simulink model "tank_based_bi_teleop_pp_kalman"  (R2020b)
settings: Solver=FixedStepAuto  StartTime=0.0  StopTime=30  FixedStep=Ts  RelTol=1e-3
values from neighbouring files (symbols this model uses):
  A = 1    [four_channel_bilateral_teleoperation_kalman_params.m]    (also in four_channel_bilateral_teleoperation_params.m; kalman_test.m = [1 Ts Ts^2/2; 0 1 Ts; 0 0 1]; recursive_estimation.m = [1 Ts Ts^2/2; 0 1 Ts; 0 0 1]; scattering_based_bi_teleop_pf_kalman_params.m)
  alpha = 0.1    [tank_based_bi_teleop_pf_kalman.m]    (also in tank_based_bi_teleop_pf_params.m; tank_based_bi_teleop_pp_kalman.m = 1; tank_based_bi_teleop_pp_params.m = 1)
  Be = 100    [four_channel_bilateral_teleoperation_architecture_params.m]    (also in four_channel_bilateral_teleoperation_kalman_params.m = 0; four_channel_bilateral_teleoperation_params.m = 0; scattering_based_bi_teleop_pf_kalman_params.m = 10; scattering_based_bi_teleop_pf_params.m = 10)
  beta = 0.01    [tank_based_bi_teleop_pf_kalman.m]    (also in tank_based_bi_teleop_pf_params.m; tank_based_bi_teleop_pp_kalman.m = 0.2; tank_based_bi_teleop_pp_params.m = 0.2)
  Bh = 70    [four_channel_bilateral_teleoperation_architecture_params.m]    (also in four_channel_bilateral_teleoperation_kalman_params.m; four_channel_bilateral_teleoperation_params.m; scattering_based_bi_teleop_pf_kalman_params.m = 1.5; scattering_based_bi_teleop_pf_params.m = 1.5)
  Bm = 1    [four_channel_bilateral_teleoperation_architecture_params.m]    (also in four_channel_bilateral_teleoperation_kalman_params.m = 0.8; four_channel_bilateral_teleoperation_params.m = 0.8; scattering_based_bi_teleop_pf_kalman_params.m = 0; scattering_based_bi_teleop_pp_kalman_params.m = 15)
  Bs = 1    [four_channel_bilateral_teleoperation_architecture_params.m]    (also in four_channel_bilateral_teleoperation_kalman_params.m = 3.2; four_channel_bilateral_teleoperation_params.m = 3.2; scattering_based_bi_teleop_pf_kalman_params.m = 40; scattering_based_bi_teleop_pf_params.m = 3)
  delay = 10    [scattering_based_bi_teleop_pf_kalman_params.m]    (also in scattering_based_bi_teleop_pf_params.m = 1; scattering_based_bi_teleop_pp_kalman_params.m = 1; scattering_based_bi_teleop_pp_params.m = 1; tank_based_bi_teleop_pf_kalman.m)
  Dm = 5    [four_channel_bilateral_teleoperation_architecture_params.m]    (also in four_channel_bilateral_teleoperation_kalman_params.m = 0; four_channel_bilateral_teleoperation_params.m = 0; scattering_based_bi_teleop_pf_kalman_params.m = 0; scattering_based_bi_teleop_pf_params.m = 0)
  Ds = 10    [four_channel_bilateral_teleoperation_architecture_params.m]    (also in four_channel_bilateral_teleoperation_kalman_params.m = 0; four_channel_bilateral_teleoperation_params.m = 0; scattering_based_bi_teleop_pf_kalman_params.m = 0; scattering_based_bi_teleop_pf_params.m = 0)
  Fc = 1    [four_channel_bilateral_teleoperation_kalman_params.m]    (also in four_channel_bilateral_teleoperation_params.m; kalman_test.m = 10; scattering_based_bi_teleop_pf_kalman_params.m = 0.1; scattering_based_bi_teleop_pf_params.m)
  Fip = 1    [four_channel_bilateral_teleoperation_kalman_params.m]    (also in four_channel_bilateral_teleoperation_params.m; scattering_based_bi_teleop_pf_kalman_params.m = 5; scattering_based_bi_teleop_pf_params.m; scattering_based_bi_teleop_pp_kalman_params.m = 5)
  h_limit = 1    [tank_based_bi_teleop_pf_kalman.m]    (also in tank_based_bi_teleop_pf_params.m = 0.5; tank_based_bi_teleop_pp_kalman.m; tank_based_bi_teleop_pp_params.m = 1.5)
  H_master_init = 1    [tank_based_bi_teleop_pf_kalman.m]    (also in tank_based_bi_teleop_pf_params.m = 0; tank_based_bi_teleop_pp_kalman.m = 5; tank_based_bi_teleop_pp_params.m = 0)
  H_slave_init = 1    [tank_based_bi_teleop_pf_kalman.m]    (also in tank_based_bi_teleop_pf_params.m = 0; tank_based_bi_teleop_pp_kalman.m = 5; tank_based_bi_teleop_pp_params.m = 0)
  Ih = 2    [scattering_based_bi_teleop_pf_kalman_params.m]    (also in scattering_based_bi_teleop_pp_kalman_params.m; tank_based_bi_teleop_pf_kalman.m; tank_based_bi_teleop_pf_params.m; tank_based_bi_teleop_pp_kalman.m)
  Je = 0    [four_channel_bilateral_teleoperation_architecture_params.m]    (also in four_channel_bilateral_teleoperation_kalman_params.m; four_channel_bilateral_teleoperation_params.m; scattering_based_bi_teleop_pf_kalman_params.m; scattering_based_bi_teleop_pf_params.m)
  Jh = 0.5    [four_channel_bilateral_teleoperation_architecture_params.m]    (also in four_channel_bilateral_teleoperation_kalman_params.m; four_channel_bilateral_teleoperation_params.m; scattering_based_bi_teleop_pf_kalman_params.m = 0; scattering_based_bi_teleop_pf_params.m = 0.05)
  Ke = 200    [four_channel_bilateral_teleoperation_architecture_params.m]    (also in four_channel_bilateral_teleoperation_kalman_params.m = 50; four_channel_bilateral_teleoperation_params.m; scattering_based_bi_teleop_pf_kalman_params.m; scattering_based_bi_teleop_pf_params.m)
  Kh = 2000    [four_channel_bilateral_teleoperation_architecture_params.m]    (also in four_channel_bilateral_teleoperation_kalman_params.m; four_channel_bilateral_teleoperation_params.m; scattering_based_bi_teleop_pf_kalman_params.m = 1; scattering_based_bi_teleop_pf_params.m = 0)
  Km = 1    [four_channel_bilateral_teleoperation_architecture_params.m]    (also in four_channel_bilateral_teleoperation_kalman_params.m; four_channel_bilateral_teleoperation_params.m; scattering_based_bi_teleop_pf_kalman_params.m = 0; scattering_based_bi_teleop_pp_kalman_params.m = 10)
  Ks = 1    [four_channel_bilateral_teleoperation_architecture_params.m]    (also in four_channel_bilateral_teleoperation_kalman_params.m = 4; four_channel_bilateral_teleoperation_params.m = 4; scattering_based_bi_teleop_pf_kalman_params.m = 50; scattering_based_bi_teleop_pf_params.m = 110)
  Mm = 0.5    [four_channel_bilateral_teleoperation_architecture_params.m]    (also in four_channel_bilateral_teleoperation_kalman_params.m; four_channel_bilateral_teleoperation_params.m; scattering_based_bi_teleop_pf_kalman_params.m; scattering_based_bi_teleop_pf_params.m)
  Ms = 2    [four_channel_bilateral_teleoperation_architecture_params.m]    (also in four_channel_bilateral_teleoperation_kalman_params.m; four_channel_bilateral_teleoperation_params.m; scattering_based_bi_teleop_pf_kalman_params.m; scattering_based_bi_teleop_pf_params.m)
  Ph = 2000    [four_channel_bilateral_teleoperation_kalman_params.m]    (also in four_channel_bilateral_teleoperation_params.m = 20100; scattering_based_bi_teleop_pf_kalman_params.m = 5; scattering_based_bi_teleop_pf_params.m = 23; scattering_based_bi_teleop_pp_kalman_params.m = 6)
  Ts = 0.001    [four_channel_bilateral_teleoperation_kalman_params.m]    (also in four_channel_bilateral_teleoperation_params.m; kalman_test.m; recursive_estimation.m; scattering_based_bi_teleop_pf_kalman_params.m)
  VarianceVelocities = 0.001    [four_channel_bilateral_teleoperation_kalman_params.m]    (also in scattering_based_bi_teleop_pf_kalman_params.m = 1e-05; scattering_based_bi_teleop_pp_kalman_params.m = 1e-05; scattering_based_bilateral_teleoperation_pp_params.m = 1e-06; tank_based_bi_teleop_pf_kalman.m = 1e-05)
settings Model: Creator=anuj  LastModifiedBy=filippo

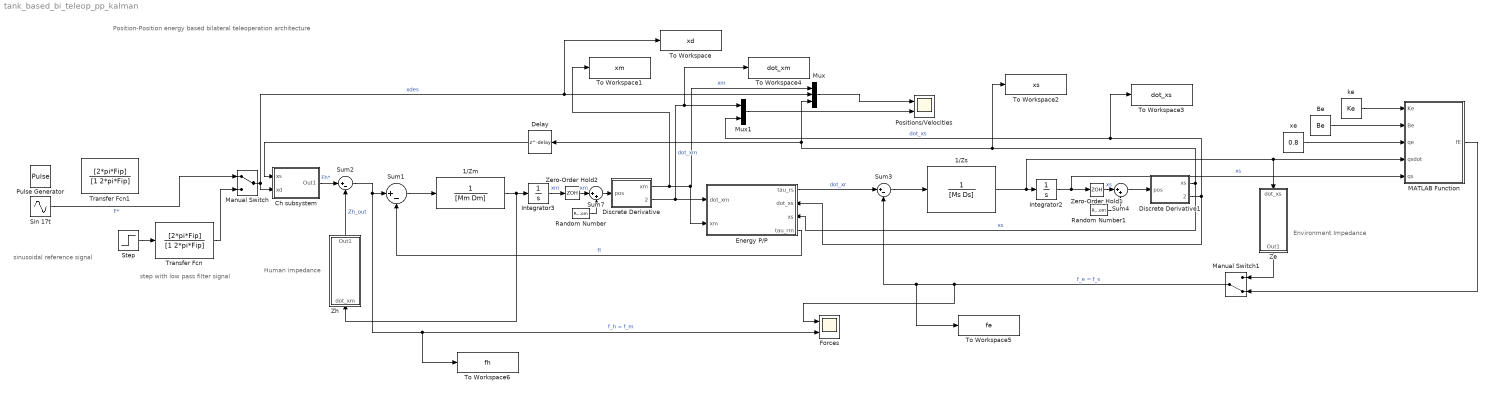
== system tank_based_bi_teleop_pp_kalman ==
  note: Position-Position energy based bilateral teleoperation architecture
  note: Environment Impedance
  note: Human impedance
  note: sinusoidal reference signal
  note: step with low pass filter signal
  1/Zm : TransferFcn  Denominator=[Mm Dm]
  1/Zs : TransferFcn  Denominator=[Ms Ds]
  Be : Constant  Value=Be
  Ch subsystem : Subsystem
  Delay : Delay  DelayLength=delay  SampleTime=Ts
  Discrete Derivative : Subsystem
  Discrete Derivative1 : Subsystem
  Energy P/P : Subsystem
      settings: PortSchema="{\"entries\":[{\"content\":{\"sides\":[{\"content\":{\"connectorIds\":[\"In1\",\"In2\"]},\"type\":\"ConnectorPlacement.EquallySpacedRectSide\",\"uuid\":\"f2b5b233-4bc9-48fa-8c02-3c8bfabc8edf\"},{\"content\":{\"connectorIds\":[\"Out1\",\"In3\",\"In4\",\"Out2\"],\"side\":\"RIGHT\"},\"type\":\"ConnectorPlacement.EquallySpacedRectSide\",\"uuid\":\"567bdcc6-c695-4210-9521-fb074471be82\"},{\"content\":{\"connectorIds\":[],\"side\":\"TOP\"},\"type\":\"ConnectorPlacement.EquallySpacedRectSide\",\"uuid\":\"1a36b9db-f8a2-44fb-9901-095b7ca2258a\"},{\"content\":{\"connectorIds\":[],\"side\":\"HIDDEN\"},\"type\":\"ConnectorPlacement.EquallySpacedRectSide\",\"uuid\":\"2e8b54c5-18c4-4c1b-a8a4-ee42e67d82c7\"}]},\"type\":\"ConnectorPlacement.EquallySpacedConnector\",\"uuid\":\"569d959e-ea5b-42c6-b188-2deb8683cad8\"}],\"packageUris\":[\"http://schema.mathworks.com/mf0/Connector/R2020b\"],\"version\":\"1.0\"}"
  Forces : Scope  NumInputPorts=2
  Integrator2 : Integrator
  Integrator3 : Integrator
  MATLAB Function : MATLAB Function  TreatAsAtomicUnit=on
  Manual Switch : ManualSwitch
  Manual Switch1 : ManualSwitch  CurrentSetting=0
  Mux : Mux  Inputs=3
  Mux1 : Mux  Inputs=2
  Positions/Velocities : Scope  NumInputPorts=2
  Pulse Generator : DiscretePulseGenerator  PulseType=Time based  Amplitude=A  PulseWidth=50  PhaseDelay=1
  Random Number : RandomNumber  Variance=VarianceVelocities  SampleTime=Ts
  Random Number1 : RandomNumber  Variance=VarianceVelocities  SampleTime=Ts
  Sin 17t : Sin  Amplitude=A  Frequency=2*pi*Fc  SampleTime=0
  Step : Step  After=A  SampleTime=0
  Sum1 : Sum  Inputs=|+-
  Sum2 : Sum  Inputs=|+-
  Sum3 : Sum  Inputs=|+-
  Sum4 : Sum  Inputs=|++
  Sum7 : Sum  Inputs=|++
  To Workspace : ToWorkspace  VariableName=xd  SaveFormat=Timeseries  SampleTime=-1
  To Workspace1 : ToWorkspace  VariableName=xm  SaveFormat=Timeseries  SampleTime=-1
  To Workspace2 : ToWorkspace  VariableName=xs  SaveFormat=Timeseries  SampleTime=-1
  To Workspace3 : ToWorkspace  VariableName=dot_xs  SaveFormat=Timeseries  SampleTime=-1
  To Workspace4 : ToWorkspace  VariableName=dot_xm  SaveFormat=Timeseries  SampleTime=-1
  To Workspace5 : ToWorkspace  VariableName=fe  SaveFormat=Timeseries  SampleTime=-1
  To Workspace6 : ToWorkspace  VariableName=fh  SaveFormat=Timeseries  SampleTime=-1
  Transfer Fcn : TransferFcn  Numerator=[2*pi*Fip]  Denominator=[1 2*pi*Fip]
  Transfer Fcn1 : TransferFcn  Numerator=[2*pi*Fip]  Denominator=[1 2*pi*Fip]
  Ze : Subsystem
  Zero-Order Hold1 : ZeroOrderHold  SampleTime=Ts
  Zero-Order Hold2 : ZeroOrderHold  SampleTime=Ts
  Zh : Subsystem
  ke : Constant  Value=Ke
  xe : Constant  Value=0.8
  wires:
  Sum2/1 -> To Workspace6/1, Forces/2, Sum1/1  "f_h = f_m"
  1/Zm/1 -> Integrator3/1, Zh/1(dot_xm)
  Sum1/1 -> 1/Zm/1
  Energy P/P/2(tau_rm) -> Sum1/2  "fl"
  Manual Switch1/1 -> Sum3/2, To Workspace5/1, Forces/1  "f_e = f_s"
  Be/1 -> MATLAB Function/2(Be)
  xe/1 -> MATLAB Function/3(qe)
  ke/1 -> MATLAB Function/1(Ke)
  Transfer Fcn/1 -> Manual Switch/2
  Step/1 -> Transfer Fcn/1
  Zh/1(Out1) -> Sum2/2  "Zh_out"
  Discrete Derivative1/2(dot_xs) -> Energy P/P/3(dot_xs), To Workspace3/1, Mux1/2  "dot_xs"
  1/Zs/1 -> Integrator2/1, Ze/1(dot_xs), MATLAB Function/4(qsdot)
  Integrator2/1 -> Zero-Order Hold1/1, MATLAB Function/5(qs)  "xs"
  Integrator3/1 -> Zero-Order Hold2/1  "xm"
  Ze/1(Out1) -> Manual Switch1/1
  MATLAB Function/1(fE) -> Manual Switch1/2
  Mux1/1 -> Positions/Velocities/2
  Mux/1 -> Positions/Velocities/1
  Manual Switch/1 -> To Workspace/1, Mux/2, Ch subsystem/2(xd)  "xdes"
  Ch subsystem/1(Out1) -> Sum2/1  "Fh*"
  Delay/1 -> Ch subsystem/1(xs)
  Sin 17t/1 -> Manual Switch/1  "F*"
  Energy P/P/1(tau_rs) -> Sum3/1  "dot_xr"
  Sum3/1 -> 1/Zs/1
  Random Number/1 -> Sum7/2
  Zero-Order Hold2/1 -> Sum7/1  "xm"
  Sum7/1 -> Discrete Derivative/1(pos)
  Random Number1/1 -> Sum4/2
  Sum4/1 -> Discrete Derivative1/1(pos)
  Zero-Order Hold1/1 -> Sum4/1  "xs"
  Discrete Derivative/2(dot_xm) -> Energy P/P/1(dot_xm), To Workspace4/1, Mux1/1  "dot_xm"
  Discrete Derivative/1(xm) -> To Workspace1/1, Energy P/P/2(xm), Mux/1  "xm"
  Discrete Derivative1/1(xs) -> Energy P/P/4(xs), To Workspace2/1, Delay/1, Mux/3  "xs"

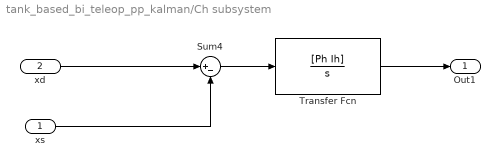
== system tank_based_bi_teleop_pp_kalman/Ch subsystem ==
  xs : Inport
  xd : Inport  Port=2
  Sum4 : Sum  Inputs=|+-
  Transfer Fcn : TransferFcn  Numerator=[Ph Ih]  Denominator=[1 0]
  Out1 : Outport
  wires:
  xd/1 -> Sum4/1
  xs/1 -> Sum4/2
  Sum4/1 -> Transfer Fcn/1
  Transfer Fcn/1 -> Out1/1

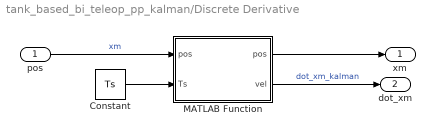
== system tank_based_bi_teleop_pp_kalman/Discrete Derivative ==
  pos : Inport
  Constant : Constant  Value=Ts
  MATLAB Function : MATLAB Function  TreatAsAtomicUnit=on
  xm : Outport
  dot_xm : Outport  Port=2
  wires:
  pos/1 -> MATLAB Function/1("pos ")  "xm"
  Constant/1 -> MATLAB Function/2(Ts)
  MATLAB Function/1(pos) -> xm/1
  MATLAB Function/2(vel) -> dot_xm/1  "dot_xm_kalman"

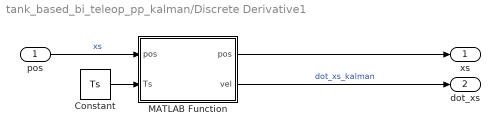
== system tank_based_bi_teleop_pp_kalman/Discrete Derivative1 ==
  pos : Inport
  Constant : Constant  Value=Ts
  MATLAB Function : MATLAB Function  TreatAsAtomicUnit=on
  xs : Outport
  dot_xs : Outport  Port=2
  wires:
  pos/1 -> MATLAB Function/1("pos ")  "xs"
  Constant/1 -> MATLAB Function/2(Ts)
  MATLAB Function/1(pos) -> xs/1
  MATLAB Function/2(vel) -> dot_xs/1  "dot_xs_kalman"

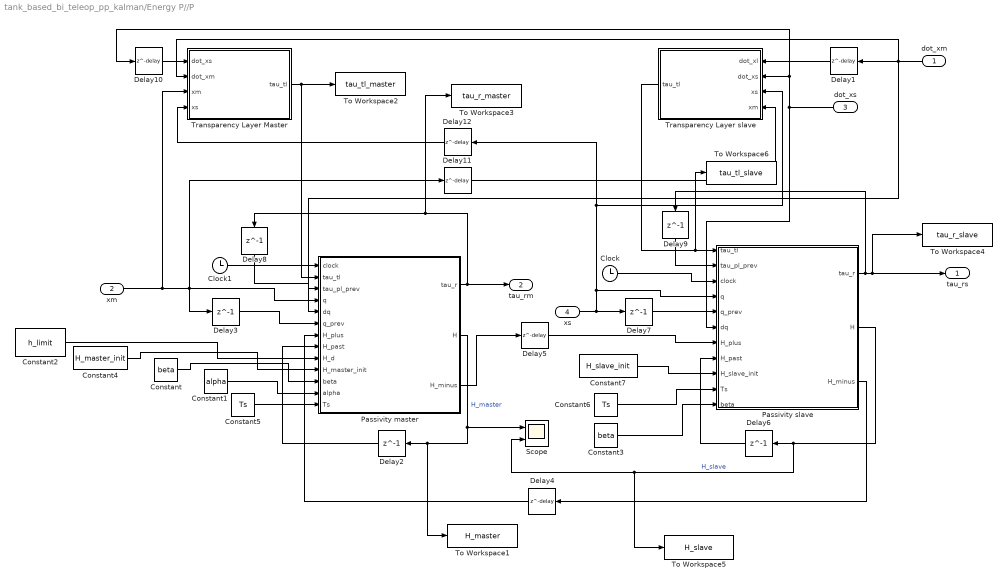
== system tank_based_bi_teleop_pp_kalman/Energy P//P ==
  dot_xm : Inport
  xm : Inport  Port=2
  dot_xs : Inport  Port=3
  xs : Inport  Port=4
  Clock : Clock
  Clock1 : Clock
  Constant : Constant  Value=beta
  Constant1 : Constant  Value=alpha
  Constant2 : Constant  Value=h_limit
  Constant3 : Constant  Value=beta
  Constant4 : Constant  Value=H_master_init
  Constant5 : Constant  Value=Ts
  Constant6 : Constant  Value=Ts
  Constant7 : Constant  Value=H_slave_init
  Delay{1,4..5,10..12} (6 alike) : Delay  DelayLength=delay  SampleTime=Ts
  Delay{2..3,6..9} (6 alike) : Delay  DelayLength=1  SampleTime=Ts
  Passivity master : MATLAB Function  TreatAsAtomicUnit=on
  Passivity slave : MATLAB Function  TreatAsAtomicUnit=on
  Scope : Scope  NumInputPorts=2
  To Workspace1 : ToWorkspace  VariableName=H_master  SaveFormat=Timeseries  SampleTime=-1
  To Workspace2 : ToWorkspace  VariableName=tau_tl_master  SaveFormat=Timeseries  SampleTime=-1
  To Workspace3 : ToWorkspace  VariableName=tau_r_master  SaveFormat=Timeseries  SampleTime=-1
  To Workspace4 : ToWorkspace  VariableName=tau_r_slave  SaveFormat=Timeseries  SampleTime=-1
  To Workspace5 : ToWorkspace  VariableName=H_slave  SaveFormat=Timeseries  SampleTime=-1
  To Workspace6 : ToWorkspace  VariableName=tau_tl_slave  SaveFormat=Timeseries  SampleTime=-1
  Transparency Layer Master : Subsystem
  Transparency Layer slave : Subsystem
  tau_rs : Outport
  tau_rm : Outport  Port=2
  wires:
  dot_xm/1 -> Passivity master/5(dq), Transparency Layer Master/2(dot_xm), Delay1/1
  Delay2/1 -> Passivity master/8(H_past)
  xm/1 -> Transparency Layer Master/3(xm), Passivity master/4(q), Delay11/1, Delay3/1
  Delay3/1 -> Passivity master/6(q_prev)
  Passivity slave/2(H) -> To Workspace5/1, Scope/2, Delay6/1  "H_slave"
  Delay4/1 -> Passivity master/7(H_plus)
  Passivity master/3(H_minus) -> Delay5/1
  Delay5/1 -> Passivity slave/7(H_plus)
  xs/1 -> Passivity slave/4(q), Transparency Layer slave/3(xs), Delay12/1, Delay7/1
  Delay6/1 -> Passivity slave/8(H_past)
  Delay7/1 -> Passivity slave/5(q_prev)
  Constant/1 -> Passivity master/11(beta)
  Constant1/1 -> Passivity master/12(alpha)
  Constant2/1 -> Passivity master/9(H_d)
  Passivity master/2(H) -> Scope/1, To Workspace1/1, Delay2/1  "H_master"
  Passivity slave/3(H_minus) -> Delay4/1
  Constant3/1 -> Passivity slave/11(beta)
  Constant4/1 -> Passivity master/10(H_master_init)
  Constant5/1 -> Passivity master/13(Ts)
  Constant6/1 -> Passivity slave/10(Ts)
  Constant7/1 -> Passivity slave/9(H_slave_init)
  Clock/1 -> Passivity slave/3(clock)
  Transparency Layer Master/1(tau_tl) -> Passivity master/2(tau_tl), To Workspace2/1
  dot_xs/1 -> Passivity slave/6(dq), Delay10/1, Transparency Layer slave/2(dot_xs)
  Delay1/1 -> Transparency Layer slave/1(dot_xl)
  Transparency Layer slave/1(tau_tl) -> To Workspace6/1, Passivity slave/1(tau_tl)
  Passivity master/1(tau_r) -> tau_rm/1, To Workspace3/1, Delay8/1
  Passivity slave/1(tau_r) -> Delay9/1, tau_rs/1, To Workspace4/1
  Delay9/1 -> Passivity slave/2(tau_pl_prev)
  Delay10/1 -> Transparency Layer Master/1(dot_xs)
  Delay11/1 -> Transparency Layer slave/4(xm)
  Delay12/1 -> Transparency Layer Master/4(xs)
  Clock1/1 -> Passivity master/1(clock)
  Delay8/1 -> Passivity master/3(tau_pl_prev)

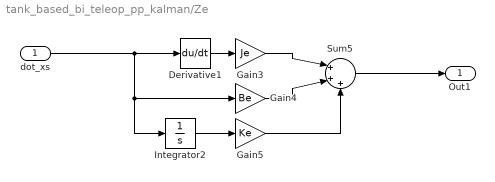
== system tank_based_bi_teleop_pp_kalman/Ze ==
  dot_xs : Inport
  Derivative1 : Derivative
  Gain3 : Gain  Gain=Je
  Gain4 : Gain  Gain=Be
  Gain5 : Gain  Gain=Ke
  Integrator2 : Integrator
  Sum5 : Sum  Inputs=|+++
  Out1 : Outport
  wires:
  Gain4/1 -> Sum5/2
  Gain3/1 -> Sum5/1
  Gain5/1 -> Sum5/3
  Sum5/1 -> Out1/1
  Integrator2/1 -> Gain5/1
  dot_xs/1 -> Integrator2/1, Gain4/1, Derivative1/1
  Derivative1/1 -> Gain3/1

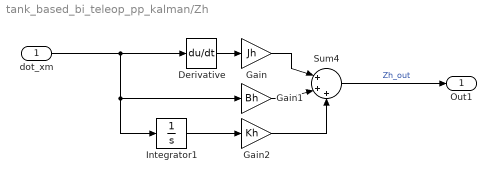
== system tank_based_bi_teleop_pp_kalman/Zh ==
  dot_xm : Inport
  Derivative : Derivative
  Gain : Gain  Gain=Jh
  Gain1 : Gain  Gain=Bh
  Gain2 : Gain  Gain=Kh
  Integrator1 : Integrator
  Sum4 : Sum  Inputs=|+++
  Out1 : Outport
  wires:
  Derivative/1 -> Gain/1
  Integrator1/1 -> Gain2/1
  Gain2/1 -> Sum4/3
  Gain1/1 -> Sum4/2
  Gain/1 -> Sum4/1
  Sum4/1 -> Out1/1  "Zh_out"
  dot_xm/1 -> Gain1/1, Integrator1/1, Derivative/1

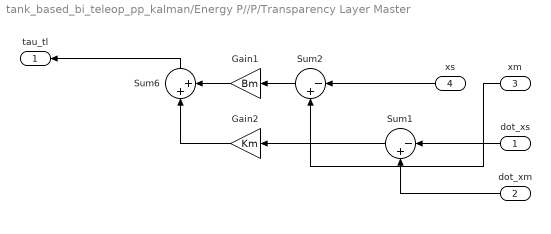
== system tank_based_bi_teleop_pp_kalman/Energy P//P/Transparency Layer Master ==
  dot_xs : Inport
  dot_xm : Inport  Port=2
  xm : Inport  Port=3
  xs : Inport  Port=4
  Gain1 : Gain  Gain=Bm
  Gain2 : Gain  Gain=Km
  Sum1 : Sum  Inputs=|-+
  Sum2 : Sum  Inputs=|-+
  Sum6 : Sum  Inputs=|++
  tau_tl : Outport
  wires:
  Sum1/1 -> Gain2/1
  Sum6/1 -> tau_tl/1
  dot_xm/1 -> Sum1/2
  Sum2/1 -> Gain1/1
  dot_xs/1 -> Sum1/1
  Gain2/1 -> Sum6/1
  Gain1/1 -> Sum6/2
  xs/1 -> Sum2/1
  xm/1 -> Sum2/2

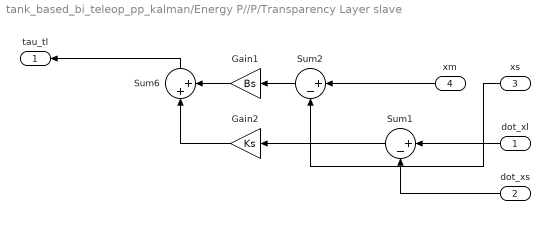
== system tank_based_bi_teleop_pp_kalman/Energy P//P/Transparency Layer slave ==
  dot_xl : Inport
  dot_xs : Inport  Port=2
  xs : Inport  Port=3
  xm : Inport  Port=4
  Gain1 : Gain  Gain=Bs
  Gain2 : Gain  Gain=Ks
  Sum1 : Sum  Inputs=|+-
  Sum2 : Sum  Inputs=|+-
  Sum6 : Sum  Inputs=|++
  tau_tl : Outport
  wires:
  Sum1/1 -> Gain2/1
  Sum6/1 -> tau_tl/1
  dot_xs/1 -> Sum1/2
  Sum2/1 -> Gain1/1
  dot_xl/1 -> Sum1/1
  Gain2/1 -> Sum6/1
  Gain1/1 -> Sum6/2
  xm/1 -> Sum2/1
  xs/1 -> Sum2/2

== matlab function tank_based_bi_teleop_pp_kalman/Energy P//P/Passivity master ==
  data: clock input; tau_tl input; tau_pl_prev input; tau_r output; q input; dq input; q_prev input; H_plus input; H_past input; H_d input; H_master_init input; beta input; alpha input; H output; H_minus output; Ts input
function [tau_r,H,H_minus] = passivity_master(clock, tau_tl, tau_pl_prev, q, dq, q_prev, H_plus, H_past, H_d, H_master_init, beta, alpha, Ts)
    if clock == 0
        H_past = H_master_init;
        tau_pl_prev = 0; 
    end
    
    % Compute energy in the tank
    delta_H = tau_pl_prev*(q - q_prev);
    H = H_past + H_plus - delta_H;

    % Computer first tau limit
    if H <= 0 
        tau_max_1 = 0;
    else
        tau_max_1 = tau_tl;
    end

    % Compute second tau limit
    if abs(dq) < 0.001
        tau_max_2 = sign(dq)*10000000;
    else
        tau_max_2 =  H/(dq*Ts);
    end

    % Compute tau_rm (Add tlc in case later)
    tau_r = sign(tau_tl)*min(abs(tau_max_1),abs(tau_max_2));

    % Use tlc if necessary
    if(H < H_d)
       d = alpha*(H_d - H);
       tau_TLC = -d*dq;
       tau_r = tau_r + tau_TLC;
    end
    
    % Send energy if possible
    H_minus = 0;
    if (H > 0)
        H_minus = beta*H;
        H = H - H_minus;  
    end
end

== matlab function tank_based_bi_teleop_pp_kalman/MATLAB Function ==
  data: Ke input; fE output; Be input; qe input; qsdot input; qs input
function fE = environment(Ke, Be, qe, qsdot, qs)
    if qs > qe
        fE = Ke * (qs - qe) + Be * qsdot; % Plot both contributions Ke and Be
    else
        fE = 0;
    end
end

== matlab function tank_based_bi_teleop_pp_kalman/Energy P//P/Passivity slave ==
  data: tau_tl input; tau_pl_prev input; clock input; tau_r output; q input; q_prev input; dq input; H_plus input; H_past input; H_slave_init input; Ts input; H output; H_minus output; beta input
function [tau_r, H, H_minus] = passivity_slave(tau_tl, tau_pl_prev, clock, q, q_prev, dq, H_plus, H_past,H_slave_init,Ts, beta)
    if clock == 0
        H_past = H_slave_init;
        tau_pl_prev = 0;
    end
    
    % Compute actual energy
    delta_H = tau_pl_prev*(q - q_prev);
    H = H_past + H_plus - delta_H;

    % Compute first tau limit
    if H <= 0 
        tau_max_1 = 0;
    else
        tau_max_1 = tau_tl;
    end

    % Compute second tau limit
    tau_max_2 = H/(dq*Ts);

    % Compute tau_rm
    tau_r = sign(tau_tl)*min(abs(tau_max_1),abs(tau_max_2));
    
    % Send energy if possible
    H_minus = 0;
    if (H > 0)
        H_minus = beta*H;
        H = H - H_minus;
    end
end

== matlab function tank_based_bi_teleop_pp_kalman/Discrete Derivative/MATLAB Function ==
  data: pos output; pos input; vel output; Ts input
function [pos, vel] = kalman(pos, Ts)
    persistent P A C Q R x_filter_old P_filter_old
    if isempty(P)
        P = 0;
        x_filter_old=[pos; 0];
        P_filter_old=0.1*eye(2);
        A=[1 Ts; 0 1];
        C=[1 0];
        q=1000000;
        Q=q*[Ts^2/2;Ts]*[Ts^2/2;Ts]';
        R=1;
    end

    % Prediction step (A priori estimation)
    x_kplus1_k = A*x_filter_old;
    P_kplus1_k = A*P_filter_old*A'+Q;

    % Compute the kalman gain
    K = P_kplus1_k * C' * inv(C * P_kplus1_k * C' + R);

    % Calculate the estimation step
    x_kplus1_kplus1 = x_kplus1_k + K *(pos - C * x_kplus1_k);
    P_kplus1_kplus1 = P_kplus1_k - P_kplus1_k * C' * inv(C * P_kplus1_k * C' + R) * C * P_kplus1_k;
    
    % Next step iteration
    x_filter_old = x_kplus1_kplus1;
    P_filter_old = P_kplus1_kplus1;
    
    pos = x_kplus1_kplus1(1,:);
    vel = x_kplus1_kplus1(2,:);
end

== matlab function tank_based_bi_teleop_pp_kalman/Discrete Derivative1/MATLAB Function ==
  data: pos output; pos input; vel output; Ts input
function [pos, vel] = kalman(pos, Ts)
    persistent P A C Q R x_filter_old P_filter_old
    if isempty(P)
        P = 0;
        x_filter_old=[pos; 0];
        P_filter_old=0.1*eye(2);
        A=[1 Ts; 0 1];
        C=[1 0];
        q=1000000;
        Q=q*[Ts^2/2;Ts]*[Ts^2/2;Ts]';
        R=1;
    end

    % Prediction step (A priori estimation)
    x_kplus1_k = A*x_filter_old;
    P_kplus1_k = A*P_filter_old*A'+Q;

    % Compute the kalman gain
    K = P_kplus1_k * C' * inv(C * P_kplus1_k * C' + R);

    % Calculate the estimation step
    x_kplus1_kplus1 = x_kplus1_k + K *(pos - C * x_kplus1_k);
    P_kplus1_kplus1 = P_kplus1_k - P_kplus1_k * C' * inv(C * P_kplus1_k * C' + R) * C * P_kplus1_k;
    
    % Next step iteration
    x_filter_old = x_kplus1_kplus1;
    P_filter_old = P_kplus1_kplus1;
    
    pos = x_kplus1_kplus1(1,:);
    vel = x_kplus1_kplus1(2,:);
end
